simulink model "UAV_SIL"  (Simulink 7.5)
settings: Solver=ode3  StartTime=0.0  StopTime=30  FixedStep=SampleTime  RelTol=1e-3
values from neighbouring files (symbols this model uses):
  IntegerTimeDelay = 2    [setup.m]
  SampleTime = 0.02    [setup.m]
undefined symbols (not defined in the file or in its folder): OperatingPoint, TrimCondition
libraries: simulink_extras x15, simulink x5, Actuator_Lib x2, NonlinearModel_Lib x1, Sensors_Lib x1
settings Model: Creator=Paul Freeman  LastModifiedBy=Andrei
settings DataIOCC: LimitDataPoints=off  SaveOutput=off  SignalLogging=off
settings DebuggingCC: StrictBusMsg=Warning
settings HardwareCC: ProdIntDivRoundTo=Zero  ProdEndianess=BigEndian  ProdHWDeviceType=Freescale->32-bit PowerPC

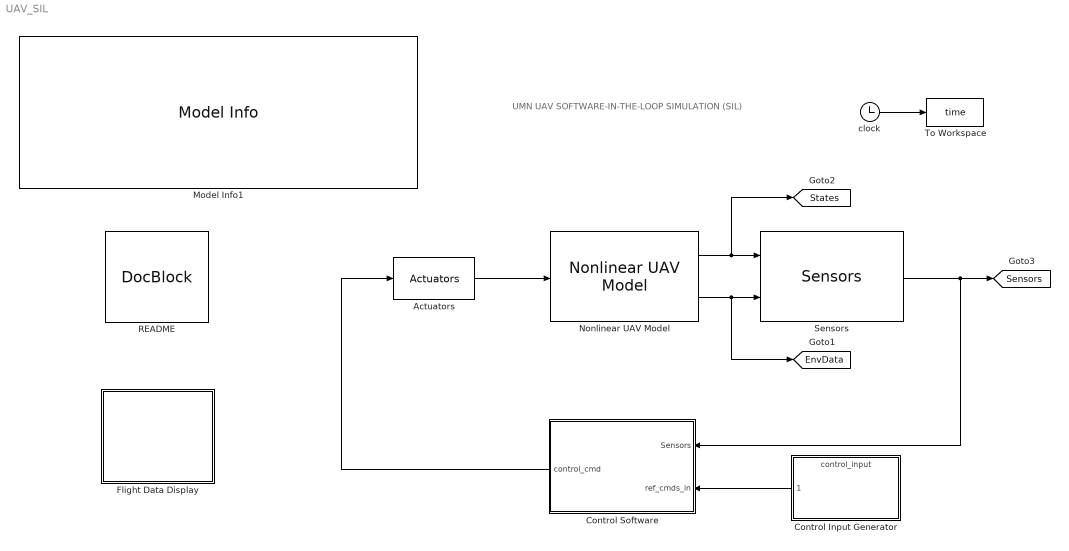
== system UAV_SIL ==
  note: UMN UAV
      | SOFTWARE-IN-THE-LOOP SIMULATION
      | (SIL)
  Actuators : Actuator_Lib/Actuators  SystemSampleTime=-1
  Control Input Generator : ModelReference  ModelNameDialog=control_input  SimulationMode=Normal  ModelReferenceVersion=1.71  CopyOfModelName=control_input
  Control Software : Subsystem
  Flight Data Display : Subsystem
      mask Display:
      | x = 0:.1:2*pi;
      | plot(x,sin(x)+rand(size(x))*.5)
  Model Info1 : simulink/Model-Wide Utilities/Model Info  SystemSampleTime=-1  InitialBlockCM=None  BlockCM=None  Frame=on  DisplayStringWithTags=|  HorizontalTextAlignment=Left  LeftAlignmentValue=0.02  SourceBlockDiagram=UAV_SIL  TagMaxNumber=20
      | MODEL INFORMATION
      | UMN UAV Software-in-the-Loop Simulation
      | 
      | University of Minnesota
      | Aerospace Engineering and Mechanics
      | Copyright 2011 Regents of the University of Minnesota. All rights reserved.
      | 
      | == SVN Info ==
      | %<ModelVersion>
      | Last modified by %<LastModifiedBy> on %<LastModificationDate>
  Nonlinear UAV Model : NonlinearModel_Lib/Nonlinear UAV Model  SystemSampleTime=-1
  README : simulink/Model-Wide Utilities/DocBlock  SystemSampleTime=-1  DocumentType=Text
  Sensors : Sensors_Lib/Sensors  SystemSampleTime=-1
  To Workspace : ToWorkspace  VariableName=time  SampleTime=-1  SaveFormat=Array
  clock : Clock
      settings: Decimation=10
  tag scope: EnvData=global, Sensors=global, States=global
  wires:
  Sensors/1 -> Control Software/1(Sensors), [Sensors]
  Nonlinear UAV Model/1 -> Sensors/1, [States]
  Nonlinear UAV Model/2 -> Sensors/2, [EnvData]
  Control Software/1(control_cmd) -> Actuators/1
  Actuators/1 -> Nonlinear UAV Model/1
  clock/1 -> To Workspace/1
  Control Input Generator/1 -> Control Software/2(ref_cmds_in)

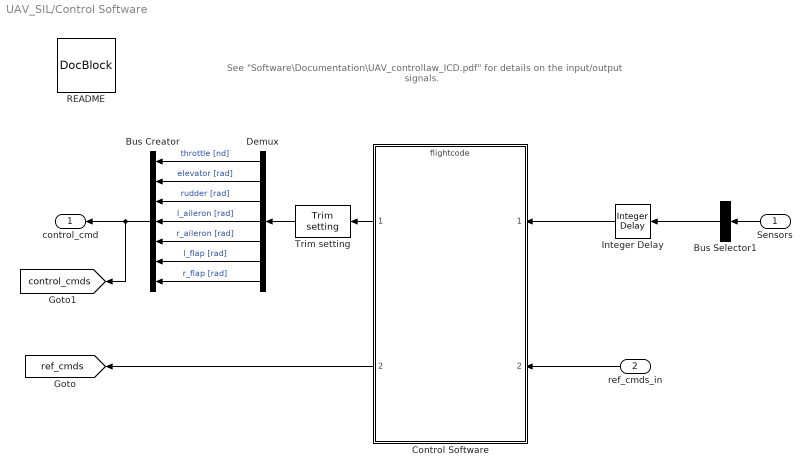
== system UAV_SIL/Control Software ==
  note: See "Software\Documentation\UAV_controllaw_ICD.pdf" for
      | details on the input/output signals.
  Sensors : Inport
  ref_cmds_in : Inport  Port=2
  Bus Creator : BusCreator  Inputs=7
  Bus Selector1 : BusSelector  OutputSignals=phi [rad],theta [rad],psi [rad],p [rad/s],q [rad/s],r [rad/s],Ax [m/s^2],Ay [m/s^2],Az [m/s^2],h [m],V_s [m/s],alpha [rad],beta [rad],Geodetic Latitude [deg],Geodetic Longitude [deg],Altitude [m],Xdot [m/s],Ydot [m/s],Zdot [m/s]  OutputAsBus=on
  Control Software : ModelReference  ModelNameDialog=flightcode  SimulationMode=Normal  Variant=on  ModelReferenceVersion=$Id$  CopyOfModelName=flightcode
  Demux : Demux  Outputs=7
  Integer Delay : simulink/Discrete/Integer Delay  vinit=repmat([TrimCondition.AttitudeIni;TrimCondition.RatesIni;TrimCondition.AccelsIni;OperatingPoint.op_report.Outputs(4).y;TrimCondition.WindAxesIni;TrimCondition.LLIni;0; zeros(3,1)],[1,IntegerTimeDelay])  samptime=-1  NumDelays=IntegerTimeDelay
  README : simulink/Model-Wide Utilities/DocBlock  SystemSampleTime=-1  DocumentType=Text
      content=|
      | Control Law Block
      |
      | This block uses Model Referencing to allow the user to easily switch out
      | control law implementations. An example usage would be first a user develops
      | a control law using simulink blocks. This controller is referred to as the
      | "simulink controller" and would be selected by setting the variable
      | "controller_mode" to 2. Once the development is completed, the user then
      | implements the Simulink controller into C-code suitable for integration
      | with the UAV software. This controller is referred to as the "flight code"
      | and would be selected by setting "controller_mode" to 1.
      |
      | This is done using the Simulink.Variant object. See the documentation for
      | more detail. The user can specify any number of variants for the Control
      | Software block; edit the ModelReferenceParameters by right-clicking this
      | block to set which Simulink model is reference for each Variant object.
      | Note that these objects must be present in the base workspace. It
      | is strongly recommended that you use the "simulink_controller.mdl" file as
      | a starting place and "Save As" to a different file name.
      |
      | In summary, to switch the Control Software, modify the "contoller_mode"
      | variable:
      | 1 = flight code controller (C implementation)
      | 2 = simulink controller (empty simulink model)
      |
      |
      | See "Software\Documentation\UAV_controllaw_ICD.pdf" for details on the
      | input/output signals.
      |
      | The control_cmd signal must have the following order:
      | throttle
      | elevator
      | rudder
      | l_aileron
      | r_aileron
      | l_flap
      | r_flap
      |
      | Control Inputs Sign Convention
      | TED = Trailing Edge Down
      | TEL = Trailing Edge Left
      | ------------------------
      | Elevator: +TED
      | Rudder: +TEL
      | Aileron: +TED, da = (da_R-da_L)/2
      | Throttle: always positive
      | Flap: +TED
      |
      |
      | The refrence command signal must have the following order:
      | 1. phi_cmd
      | 2. theta_cmd
      | 3. psi_cmd
      | 4. p_cmd
      | 5. q_cmd
      | 6. r_cmd
      | 7. V_s_cmd
      | 8. h_cmd
      | 9. gndtrk_cmd
      | 10. aoa_cmd
      | 11. aos_cmd
      | 12. gamma_cmd
      | Note the trimmed value of pitch angle theta is included in the reference
      | command. Use the Doublet Generator block (or other signal generating block)
      | to input reference commands to the Control Software.
  "Trim setting " : Actuator_Lib/Trim setting   SystemSampleTime=-1
  control_cmd : Outport
  tag scope: control_cmds=global, ref_cmds=global
  wires:
  Control Software/1 -> "Trim setting "/1
  Sensors/1 -> Bus Selector1/1
  ref_cmds_in/1 -> Control Software/2
  Bus Creator/1 -> control_cmd/1, [control_cmds]
  Demux/1 -> Bus Creator/1  "throttle [nd]"
  Demux/2 -> Bus Creator/2  "elevator [rad]"
  Demux/3 -> Bus Creator/3  "rudder [rad]"
  Demux/4 -> Bus Creator/4  "l_aileron [rad]"
  Demux/5 -> Bus Creator/5  "r_aileron [rad]"
  Demux/6 -> Bus Creator/6  "l_flap [rad]"
  Demux/7 -> Bus Creator/7  "r_flap [rad]"
  Integer Delay/1 -> Control Software/1
  Bus Selector1/1 -> Integer Delay/1
  "Trim setting "/1 -> Demux/1
  Control Software/2 -> [ref_cmds]

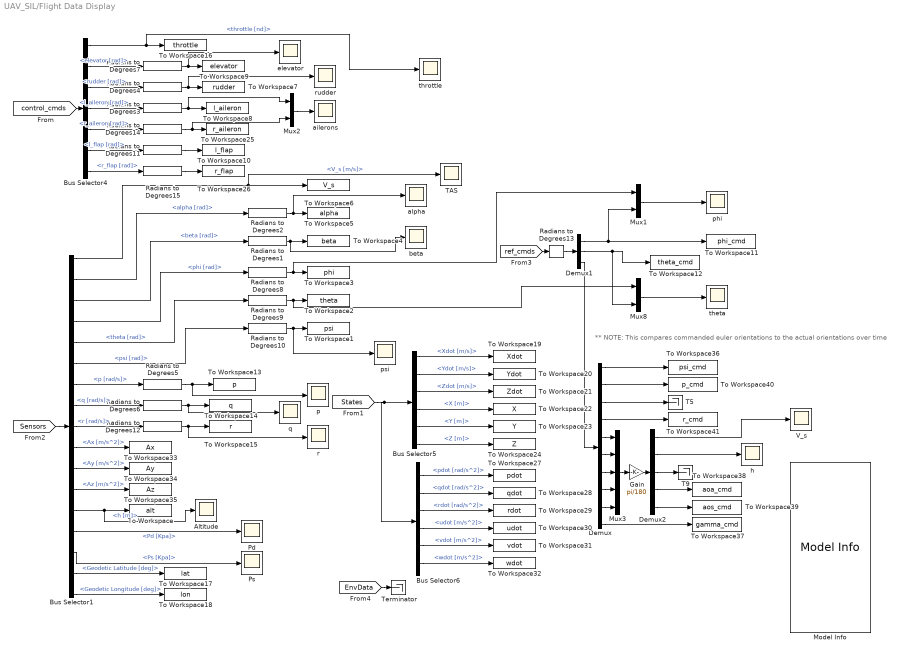
== system UAV_SIL/Flight Data Display ==
  note: ** NOTE: This compares commanded euler orientations to the actual orientations over time
  Altitude : Scope
      settings: TimeRange=60  YMin=75  YMax=115  SaveName=ScopeData10
  Bus Selector1 : BusSelector  OutputSignals=V_s [m/s],alpha [rad],beta [rad],phi [rad],theta [rad],psi [rad],p [rad/s],q [rad/s],r [rad/s],Ax [m/s^2],Ay [m/s^2],Az [m/s^2],h [m],Pd [Kpa],Ps [Kpa],Geodetic Latitude [deg],Geodetic Longitude [deg]
  Bus Selector4 : BusSelector  OutputSignals=throttle [nd],elevator [rad],rudder [rad],l_aileron [rad],r_aileron [rad],l_flap [rad],r_flap [rad]
  Bus Selector5 : BusSelector  OutputSignals=V_e [m/s].Xdot [m/s],V_e [m/s].Ydot [m/s],V_e [m/s].Zdot [m/s],X_e [m].X [m],X_e [m].Y [m],X_e [m].Z [m]
  Bus Selector6 : BusSelector  OutputSignals=AngAccel [rad/s^2].pdot [rad/s^2],AngAccel [rad/s^2].qdot [rad/s^2],AngAccel [rad/s^2].rdot [rad/s^2],A_b [m/s^2].udot [m/s^2],A_b [m/s^2].vdot [m/s^2],A_b [m/s^2].wdot [m/s^2]
  Demux : Demux  Outputs=10
  Demux1 : Demux  Outputs=[1 1 10]
  Demux2 : Demux  Outputs=5
  Gain : Gain  Gain=pi/180  ParameterDataType=fixdt(1, 16)  ParameterScaling=2^0  OutDataType=fixdt(1, 16)  OutScaling=2^0  SampleTime=SampleTime
  Model Info : simulink/Model-Wide Utilities/Model Info  SystemSampleTime=-1  InitialBlockCM=None  BlockCM=None  Frame=on  DisplayStringWithTags=|  HorizontalTextAlignment=Center  LeftAlignmentValue=0.5  SourceBlockDiagram=UAV_SIL  TagMaxNumber=20
      | Ref Cmd Port Info
      | 
      | 1. phi_cmd
      | 2. theta_cmd
      | 3. psi_cmd
      | 4. p_cmd
      | 5. q_cmd
      | 6. r_cmd
      | 7. V_s_cmd
      | 8. h_cmd
      | 9. gndtrk_cmd
      | 10. aoa_cmd
      | 11. aos_cmd
      | 12. gamma_cmd
  Mux1 : Mux  Inputs=2
  Mux2 : Mux  Inputs=2
  Mux3 : Mux  Inputs=5
  Mux8 : Mux  Inputs=2
  Pd : Scope
      settings: TimeRange=25  YMin=0.14  YMax=0.2  SaveName=ScopeData5
  Ps : Scope
      settings: TimeRange=25  YMin=100.45  YMax=100.52  SaveName=ScopeData6
  Radians to Degrees{1..15} (15 alike) : simulink_extras/Transformations/Radians to Degrees  SystemSampleTime=-1
  T5 : Terminator
  T9 : Terminator
  TAS : Scope
      settings: TimeRange=45  YMin=14  YMax=19  SaveName=ScopeData3
  Terminator : Terminator
  To Workspace : ToWorkspace  VariableName=alt  SampleTime=-1  SaveFormat=Array
  To Workspace1 : ToWorkspace  VariableName=psi  SampleTime=-1  SaveFormat=Array
  To Workspace10 : ToWorkspace  VariableName=l_flap  SampleTime=-1  SaveFormat=Array
  To Workspace11 : ToWorkspace  VariableName=phi_cmd  SampleTime=-1  SaveFormat=Array
  To Workspace12 : ToWorkspace  VariableName=theta_cmd  SampleTime=-1  SaveFormat=Array
  To Workspace13 : ToWorkspace  VariableName=p  SampleTime=-1  SaveFormat=Array
  To Workspace14 : ToWorkspace  VariableName=q  SampleTime=-1  SaveFormat=Array
  To Workspace15 : ToWorkspace  VariableName=r  SampleTime=-1  SaveFormat=Array
  To Workspace16 : ToWorkspace  VariableName=throttle  SampleTime=-1  SaveFormat=Array
  To Workspace17 : ToWorkspace  VariableName=lat  SampleTime=-1  SaveFormat=Array
  To Workspace18 : ToWorkspace  VariableName=lon  SampleTime=-1  SaveFormat=Array
  To Workspace19 : ToWorkspace  VariableName=Xdot  SampleTime=-1  SaveFormat=Array
  To Workspace2 : ToWorkspace  VariableName=theta  SampleTime=-1  SaveFormat=Array
  To Workspace20 : ToWorkspace  VariableName=Ydot  SampleTime=-1  SaveFormat=Array
  To Workspace21 : ToWorkspace  VariableName=Zdot  SampleTime=-1  SaveFormat=Array
  To Workspace22 : ToWorkspace  VariableName=X  SampleTime=-1  SaveFormat=Array
  To Workspace23 : ToWorkspace  VariableName=Y  SampleTime=-1  SaveFormat=Array
  To Workspace24 : ToWorkspace  VariableName=Z  SampleTime=-1  SaveFormat=Array
  To Workspace25 : ToWorkspace  VariableName=r_aileron  SampleTime=-1  SaveFormat=Array
  To Workspace26 : ToWorkspace  VariableName=r_flap  SampleTime=-1  SaveFormat=Array
  To Workspace27 : ToWorkspace  VariableName=pdot  SampleTime=-1  SaveFormat=Array
  To Workspace28 : ToWorkspace  VariableName=qdot  SampleTime=-1  SaveFormat=Array
  To Workspace29 : ToWorkspace  VariableName=rdot  SampleTime=-1  SaveFormat=Array
  To Workspace3 : ToWorkspace  VariableName=phi  SampleTime=-1  SaveFormat=Array
  To Workspace30 : ToWorkspace  VariableName=udot  SampleTime=-1  SaveFormat=Array
  To Workspace31 : ToWorkspace  VariableName=vdot  SampleTime=-1  SaveFormat=Array
  To Workspace32 : ToWorkspace  VariableName=wdot  SampleTime=-1  SaveFormat=Array
  To Workspace33 : ToWorkspace  VariableName=Ax  SampleTime=-1  SaveFormat=Array
  To Workspace34 : ToWorkspace  VariableName=Ay  SampleTime=-1  SaveFormat=Array
  To Workspace35 : ToWorkspace  VariableName=Az  SampleTime=-1  SaveFormat=Array
  To Workspace36 : ToWorkspace  VariableName=psi_cmd  SampleTime=-1  SaveFormat=Array
  To Workspace37 : ToWorkspace  VariableName=gamma_cmd  SampleTime=-1  SaveFormat=Array
  To Workspace38 : ToWorkspace  VariableName=aoa_cmd  SampleTime=-1  SaveFormat=Array
  To Workspace39 : ToWorkspace  VariableName=aos_cmd  SampleTime=-1  SaveFormat=Array
  To Workspace4 : ToWorkspace  VariableName=beta  SampleTime=-1  SaveFormat=Array
  To Workspace40 : ToWorkspace  VariableName=p_cmd  SampleTime=-1  SaveFormat=Array
  To Workspace41 : ToWorkspace  VariableName=r_cmd  SampleTime=-1  SaveFormat=Array
  To Workspace5 : ToWorkspace  VariableName=alpha  SampleTime=-1  SaveFormat=Array
  To Workspace6 : ToWorkspace  VariableName=V_s  SampleTime=-1  SaveFormat=Array
  To Workspace7 : ToWorkspace  VariableName=rudder  SampleTime=-1  SaveFormat=Array
  To Workspace8 : ToWorkspace  VariableName=l_aileron  SampleTime=-1  SaveFormat=Array
  To Workspace9 : ToWorkspace  VariableName=elevator  SampleTime=-1  SaveFormat=Array
  V_s : Scope
      settings: TimeRange=20  YMin=-4  YMax=10  SaveName=ScopeData16
  ailerons : Scope
      settings: TimeRange=20  YMin=-20  YMax=20  SaveName=ScopeData2
  alpha : Scope
      settings: TimeRange=25  YMin=0.035  YMax=0.08  SaveName=ScopeData7
  beta : Scope
      settings: TimeRange=25  YMin=-0.06  YMax=0.06  SaveName=ScopeData11
  elevator : Scope
      settings: TimeRange=45  YMin=4  YMax=6.5
  h : Scope
      settings: TimeRange=20  YMin=-4  YMax=10  SaveName=ScopeData18
  p : Scope
      settings: TimeRange=45  YMin=-60  YMax=30  SaveName=ScopeData8
  phi : Scope
      settings: TimeRange=20  YMin=-25  YMax=25  SaveName=ScopeData14
  psi : Scope
      settings: TimeRange=20  YMin=85  YMax=185  SaveName=ScopeData12
  q : Scope
      settings: TimeRange=45  YMax=4  SaveName=ScopeData9
  r : Scope
      settings: TimeRange=45  YMin=-8  YMax=8
  rudder : Scope
      settings: TimeRange=45  YMin=-1.5  YMax=2  SaveName=ScopeData4
  theta : Scope
      settings: TimeRange=20  YMin=-4  YMax=10  SaveName=ScopeData13
  throttle : Scope
      settings: TimeRange=25  YMin=0.4  YMax=0.75  SaveName=ScopeData15
  wires:
  Bus Selector1/1 -> To Workspace6/1, TAS/1  "<V_s [m/s]>"
  Bus Selector1/2 -> Radians to Degrees2/1  "<alpha [rad]>"
  Radians to Degrees2/1 -> To Workspace5/1, alpha/1
  Bus Selector1/3 -> Radians to Degrees1/1  "<beta [rad]>"
  Radians to Degrees1/1 -> To Workspace4/1, beta/1
  Bus Selector1/4 -> Radians to Degrees8/1  "<phi [rad]>"
  Radians to Degrees8/1 -> To Workspace3/1, Mux1/1
  Bus Selector1/5 -> Radians to Degrees9/1  "<theta [rad]>"
  Radians to Degrees9/1 -> To Workspace2/1, Mux8/1
  Bus Selector1/6 -> Radians to Degrees10/1  "<psi [rad]>"
  Radians to Degrees10/1 -> To Workspace1/1, psi/1
  Radians to Degrees3/1 -> To Workspace8/1, Mux2/1
  Radians to Degrees7/1 -> To Workspace9/1, elevator/1
  Radians to Degrees4/1 -> To Workspace7/1, rudder/1
  Radians to Degrees11/1 -> To Workspace10/1
  [ref_cmds] -> Radians to Degrees13/1
  Radians to Degrees5/1 -> To Workspace13/1, p/1
  Radians to Degrees6/1 -> To Workspace14/1, q/1
  Radians to Degrees12/1 -> To Workspace15/1, r/1
  [States] -> Bus Selector5/1, Bus Selector6/1
  Bus Selector5/1 -> To Workspace19/1  "<Xdot [m/s]>"
  Bus Selector5/2 -> To Workspace20/1  "<Ydot [m/s]>"
  Bus Selector5/3 -> To Workspace21/1  "<Zdot [m/s]>"
  Bus Selector5/4 -> To Workspace22/1  "<X [m]>"
  Bus Selector5/5 -> To Workspace23/1  "<Y [m]>"
  Bus Selector5/6 -> To Workspace24/1  "<Z [m]>"
  Radians to Degrees13/1 -> Demux1/1
  Demux1/1 -> To Workspace11/1, Mux1/2
  Bus Selector4/1 -> To Workspace16/1, throttle/1  "<throttle [nd]>"
  Bus Selector4/2 -> Radians to Degrees7/1  "<elevator [rad]>"
  Bus Selector4/3 -> Radians to Degrees4/1  "<rudder [rad]>"
  Bus Selector4/4 -> Radians to Degrees3/1  "<l_aileron [rad]>"
  Radians to Degrees14/1 -> To Workspace25/1, Mux2/2
  Bus Selector4/5 -> Radians to Degrees14/1  "<r_aileron [rad]>"
  Bus Selector4/6 -> Radians to Degrees11/1  "<l_flap [rad]>"
  Radians to Degrees15/1 -> To Workspace26/1
  Bus Selector4/7 -> Radians to Degrees15/1  "<r_flap [rad]>"
  Mux2/1 -> ailerons/1
  Bus Selector6/1 -> To Workspace27/1  "<pdot [rad/s^2]>"
  Bus Selector6/2 -> To Workspace28/1  "<qdot [rad/s^2]>"
  Bus Selector6/3 -> To Workspace29/1  "<rdot [rad/s^2]>"
  Bus Selector6/4 -> To Workspace30/1  "<udot [m/s^2]>"
  Bus Selector6/5 -> To Workspace31/1  "<vdot [m/s^2]>"
  Bus Selector6/6 -> To Workspace32/1  "<wdot [m/s^2]>"
  [control_cmds] -> Bus Selector4/1
  [Sensors] -> Bus Selector1/1
  Bus Selector1/7 -> Radians to Degrees5/1  "<p [rad/s]>"
  Bus Selector1/8 -> Radians to Degrees6/1  "<q [rad/s]>"
  Bus Selector1/9 -> Radians to Degrees12/1  "<r [rad/s]>"
  Bus Selector1/10 -> To Workspace33/1  "<Ax [m/s^2]>"
  Bus Selector1/11 -> To Workspace34/1  "<Ay [m/s^2]>"
  Bus Selector1/12 -> To Workspace35/1  "<Az [m/s^2]>"
  Bus Selector1/13 -> To Workspace/1, Altitude/1  "<h [m]>"
  Bus Selector1/14 -> Pd/1  "<Pd [Kpa]>"
  Bus Selector1/15 -> Ps/1  "<Ps [Kpa]>"
  Bus Selector1/16 -> To Workspace17/1  "<Geodetic Latitude [deg]>"
  Bus Selector1/17 -> To Workspace18/1  "<Geodetic Longitude [deg]>"
  [EnvData] -> Terminator/1
  Demux/1 -> To Workspace36/1
  Demux/3 -> T5/1
  Demux/4 -> To Workspace41/1
  Demux/6 -> Mux3/2
  Demux/5 -> Mux3/1
  Demux/7 -> Mux3/3
  Demux2/3 -> T9/1
  Demux2/1 -> V_s/1
  Demux2/2 -> h/1
  Mux1/1 -> phi/1
  Demux1/3 -> Demux/1
  Demux/8 -> Mux3/4
  Demux/9 -> Mux3/5
  Demux2/4 -> To Workspace38/1
  Demux2/5 -> To Workspace39/1
  Demux/2 -> To Workspace40/1
  Demux/10 -> To Workspace37/1
  Mux3/1 -> Gain/1
  Gain/1 -> Demux2/1
  Mux8/1 -> theta/1
  Demux1/2 -> To Workspace12/1, Mux8/2
